simulink model "gtcs_math_magnetic_v0"  (R2022a)
settings: Solver=FixedStepDiscrete  StartTime=0.0  StopTime=10  FixedStep=1e-05  RelTol=1e-3
values from neighbouring files (symbols this model uses):
  B_r = 0.0001    [gtcs_math_magnetic_v0_dd.sldd]    (also in gtcs_math_magnetic_v0_parameter.mat)
  current_lim = 40.0    [gtcs_math_magnetic_v0_dd.sldd]    (also in gtcs_math_magnetic_v0_parameter.mat = 40)
  J_r = 0.00025    [gtcs_math_magnetic_v0_dd.sldd]    (also in gtcs_math_magnetic_v0_parameter.mat)
  L = 6.0E-6    [gtcs_math_magnetic_v0_dd.sldd]    (also in gtcs_math_magnetic_v0_parameter.mat = 6e-06)
  M = 3.0E-6    [gtcs_math_magnetic_v0_dd.sldd]    (also in gtcs_math_magnetic_v0_parameter.mat = 3e-06)
  P = 1.0    [gtcs_math_magnetic_v0_dd.sldd]    (also in gtcs_math_magnetic_v0_parameter.mat = 1)
  phase_a = 0.0    [gtcs_math_magnetic_v0_dd.sldd]    (also in gtcs_math_magnetic_v0_parameter.mat = 0)
  phase_b = 2.0943951023931953    [gtcs_math_magnetic_v0_dd.sldd]    (also in gtcs_math_magnetic_v0_parameter.mat = 2.09439510239)
  phase_c = -2.0943951023931953    [gtcs_math_magnetic_v0_dd.sldd]    (also in gtcs_math_magnetic_v0_parameter.mat = -2.09439510239)
  Phi_m = 0.04    [gtcs_math_magnetic_v0_dd.sldd]    (also in gtcs_math_magnetic_v0_parameter.mat)
  R = 0.015    [gtcs_math_magnetic_v0_dd.sldd]    (also in gtcs_math_magnetic_v0_parameter.mat)
undefined symbols (not defined in the file or in its folder): DiscIntNeverNeededParam
libraries: simulink x3
settings Model: DataDictionary=gtcs_math_magnetic_v0_dd.sldd  Creator=yusuf.ogut  LastModifiedBy=yusuf.ogut

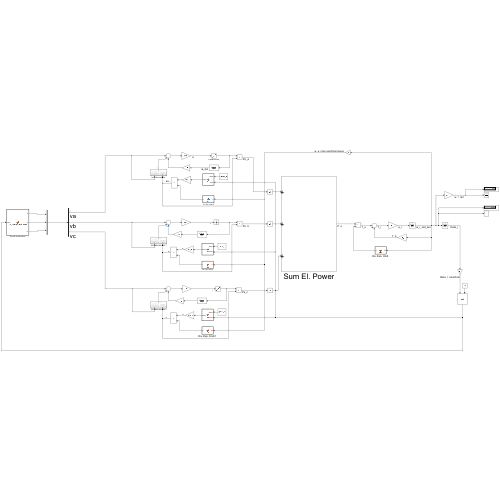
[thumbnail: Simulink's stored preview of the top-level diagram]
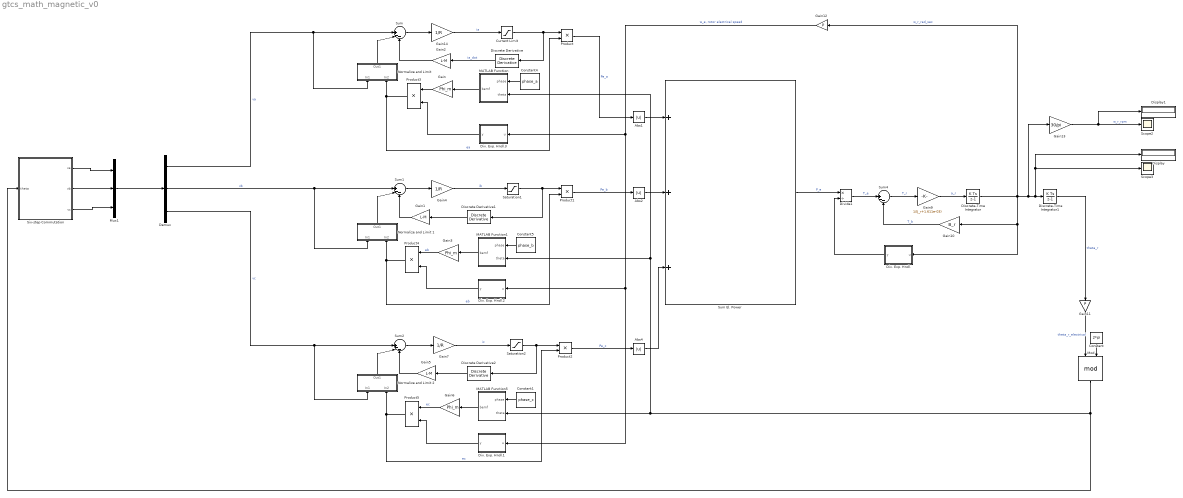
== system gtcs_math_magnetic_v0 ==
  Abs1 : Abs  SaturateOnIntegerOverflow=off
  Abs2 : Abs  SaturateOnIntegerOverflow=off
  Abs4 : Abs  SaturateOnIntegerOverflow=off
  Constant : Constant  Value=2*pi
  Constant1 : Constant  Value=phase_c
  Constant4 : Constant  Value=phase_a
  Constant5 : Constant  Value=phase_b
  Current Limit : Saturate  UpperLimit=current_lim  LowerLimit=-current_lim
  Demux : Demux  Outputs=3
  Discrete Derivative : simulink/Discrete/Discrete Derivative  gainval=1.0  ICPrevScaledInput=0.0  OutMin=[]  OutMax=[]  OutDataType=fixdt(1, 16)  OutScaling=2^-10  DoSatur=off
  Discrete Derivative1 : simulink/Discrete/Discrete Derivative  gainval=1.0  ICPrevScaledInput=0.0  OutMin=[]  OutMax=[]  OutDataType=fixdt(1, 16)  OutScaling=2^-10  DoSatur=off
  Discrete Derivative2 : simulink/Discrete/Discrete Derivative  gainval=1.0  ICPrevScaledInput=0.0  OutMin=[]  OutMax=[]  OutDataType=fixdt(1, 16)  OutScaling=2^-10  DoSatur=off
  Discrete-Time Integrator : DiscreteIntegrator  SampleTime=-1  ICPrevOutput=DiscIntNeverNeededParam  ICPrevScaledInput=DiscIntNeverNeededParam
  Discrete-Time Integrator1 : DiscreteIntegrator  SampleTime=-1  ICPrevOutput=DiscIntNeverNeededParam  ICPrevScaledInput=DiscIntNeverNeededParam
  Display : Display
  Display1 : Display
  Div. Exp. Hndl. : MATLAB Function  TreatAsAtomicUnit=on
  Div. Exp. Hndl.1 : MATLAB Function  TreatAsAtomicUnit=on
  Div. Exp. Hndl.2 : MATLAB Function  TreatAsAtomicUnit=on
  Div. Exp. Hndl.3 : MATLAB Function  TreatAsAtomicUnit=on
  Divide1 : Product  Inputs=*/
  Gain : Gain  Gain=Phi_m
  Gain1 : Gain  Gain=L-M
  Gain10 : Gain  Gain=B_r
  Gain11 : Gain  Gain=P
  Gain12 : Gain  Gain=P
  Gain13 : Gain  Gain=30/pi
  Gain14 : Gain  Gain=1/R
  Gain2 : Gain  Gain=L-M
  Gain3 : Gain  Gain=Phi_m
  Gain4 : Gain  Gain=1/R
  Gain5 : Gain  Gain=L-M
  Gain6 : Gain  Gain=Phi_m
  Gain7 : Gain  Gain=1/R
  Gain9 : Gain  Gain=1/(J_r+1.611e-03)
  MATLAB Function : MATLAB Function  TreatAsAtomicUnit=on
  MATLAB Function1 : MATLAB Function  TreatAsAtomicUnit=on
  MATLAB Function5 : MATLAB Function  TreatAsAtomicUnit=on
  Mod : Math  Operator=mod
  Mux1 : Mux  Inputs=3
  Normalize and Limit : Subsystem
  Normalize and Limit 1 : Subsystem
  Normalize and Limit 2 : Subsystem
  Product{,1..5} (6 alike) : Product
  Saturation1 : Saturate  UpperLimit=current_lim  LowerLimit=-current_lim
  Saturation2 : Saturate  UpperLimit=current_lim  LowerLimit=-current_lim
  Scope2 : Scope
  Scope3 : Scope
  Six-step Commutation : MATLAB Function  TreatAsAtomicUnit=on
  Sum{,1..2,4} (4 alike) : Sum  Inputs=||+--
  Sum El. Power : Sum  Inputs=+++
  wires:
  Demux/1 -> Sum/1, Normalize and Limit/1(In1)  "va"
  Gain14/1 -> Current Limit/1  "ia"
  Discrete Derivative/1 -> Gain2/1  "ia_dot"
  Product3/1 -> Normalize and Limit/2(In2), Product/2  "ea"
  Constant4/1 -> MATLAB Function/1(phase)
  Gain4/1 -> Saturation1/1  "ib"
  Constant5/1 -> MATLAB Function1/1(phase)
  Gain1/1 -> Sum1/3
  MATLAB Function1/1(bemf) -> Gain3/1
  Product4/1 -> Product1/2, Normalize and Limit 1/2(In2)  "eb"
  Demux/2 -> Sum1/1, Normalize and Limit 1/1(In1)  "vb"
  Sum1/1 -> Gain4/1
  Discrete Derivative1/1 -> Gain1/1
  MATLAB Function5/1(bemf) -> Gain6/1
  Demux/3 -> Sum2/1, Normalize and Limit 2/1(In1)  "vc"
  Product5/1 -> Normalize and Limit 2/2(In2), Product2/2  "ec"
  Discrete Derivative2/1 -> Gain5/1
  Gain5/1 -> Sum2/3
  Sum2/1 -> Gain7/1
  Gain7/1 -> Saturation2/1  "ic"
  Constant1/1 -> MATLAB Function5/1(phase)
  Sum4/1 -> Gain9/1  "T_r"
  Gain9/1 -> Discrete-Time Integrator/1  "a_r"
  Gain10/1 -> Sum4/3  "T_b"
  Discrete-Time Integrator/1 -> Gain12/1, Gain13/1, Scope3/1, Display/1, Discrete-Time Integrator1/1, Div. Exp. Hndl./1(u), Gain10/1  "w_r_rad_sec"
  Discrete-Time Integrator1/1 -> Gain11/1  "theta_r"
  Sum El. Power/1 -> Divide1/1  "P_e"
  Gain11/1 -> Mod/1  "theta_r_electrical"
  Constant/1 -> Mod/2
  Div. Exp. Hndl./1(y) -> Divide1/2
  Product/1 -> Abs1/1  "Pe_a"
  Divide1/1 -> Sum4/1  "T_e"
  Saturation1/1 -> Product1/1, Discrete Derivative1/1
  Saturation2/1 -> Discrete Derivative2/1, Product2/1
  Six-step Commutation/3(vc) -> Mux1/3
  Six-step Commutation/2(vb) -> Mux1/2
  Six-step Commutation/1(va) -> Mux1/1
  Mux1/1 -> Demux/1
  Gain12/1 -> Div. Exp. Hndl.3/1(u), Div. Exp. Hndl.1/1(u), Div. Exp. Hndl.2/1(u)  "w_e, rotor electrical speed"
  Gain/1 -> Product3/1
  Gain3/1 -> Product4/1  "eb"
  Gain6/1 -> Product5/1  "ec"
  Div. Exp. Hndl.3/1(y) -> Product3/2
  Div. Exp. Hndl.2/1(y) -> Product4/2
  Div. Exp. Hndl.1/1(y) -> Product5/2
  Gain13/1 -> Display1/1, Scope2/1  "w_r_rpm"
  Product1/1 -> Abs2/1  "Pe_b"
  Product2/1 -> Abs4/1  "Pe_c"
  Current Limit/1 -> Product/1, Discrete Derivative/1
  Normalize and Limit 1/1(Out1) -> Sum1/2
  Normalize and Limit 2/1(Out1) -> Sum2/2
  Normalize and Limit/1(Out1) -> Sum/2
  Sum/1 -> Gain14/1
  Abs1/1 -> Sum El. Power/1
  Abs2/1 -> Sum El. Power/2
  Mod/1 -> MATLAB Function5/2(theta), MATLAB Function1/2(theta), MATLAB Function/2(theta), Six-step Commutation/1(theta)
  Abs4/1 -> Sum El. Power/3
  Gain2/1 -> Sum/3
  MATLAB Function/1(bemf) -> Gain/1

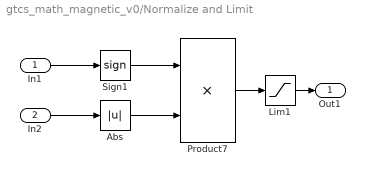
== system gtcs_math_magnetic_v0/Normalize and Limit ==
  In1 : Inport
  In2 : Inport  Port=2
  Abs : Abs  SaturateOnIntegerOverflow=off
  Lim1 : Saturate  UpperLimit=28  LowerLimit=-28
  Product7 : Product
  Sign1 : Signum
  Out1 : Outport
  wires:
  Lim1/1 -> Out1/1
  In2/1 -> Abs/1
  Sign1/1 -> Product7/1
  In1/1 -> Sign1/1
  Product7/1 -> Lim1/1
  Abs/1 -> Product7/2

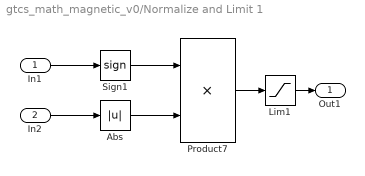
== system gtcs_math_magnetic_v0/Normalize and Limit 1 ==
  In1 : Inport
  In2 : Inport  Port=2
  Abs : Abs  SaturateOnIntegerOverflow=off
  Lim1 : Saturate  UpperLimit=28  LowerLimit=-28
  Product7 : Product
  Sign1 : Signum
  Out1 : Outport
  wires:
  Abs/1 -> Product7/2
  Product7/1 -> Lim1/1
  In1/1 -> Sign1/1
  Sign1/1 -> Product7/1
  In2/1 -> Abs/1
  Lim1/1 -> Out1/1

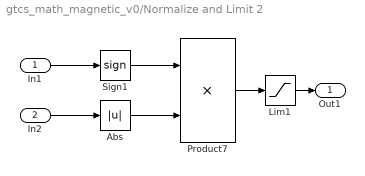
== system gtcs_math_magnetic_v0/Normalize and Limit 2 ==
  In1 : Inport
  In2 : Inport  Port=2
  Abs : Abs  SaturateOnIntegerOverflow=off
  Lim1 : Saturate  UpperLimit=28  LowerLimit=-28
  Product7 : Product
  Sign1 : Signum
  Out1 : Outport
  wires:
  Lim1/1 -> Out1/1
  In2/1 -> Abs/1
  Sign1/1 -> Product7/1
  In1/1 -> Sign1/1
  Product7/1 -> Lim1/1
  Abs/1 -> Product7/2

== matlab function gtcs_math_magnetic_v0/MATLAB Function ==
  data: phase input; bemf output; theta input
function bemf = fcn(phase, theta)
    theta_temp = mod(theta - phase,2*pi); % minus??
    bemf = 0;
    if theta_temp>=0 && theta_temp<(pi/6)
        %bemf = -theta_temp/(pi/6);
        bemf = -1;
    elseif theta_temp>=(pi/6) && theta_temp<(5*pi/6)
        bemf = -1;
    elseif theta_temp>=(5*pi/6) && theta_temp<(pi)
        %bemf = -1 + (theta_temp-5*pi/6)/(pi-5*pi/6);
        bemf = -1;
    elseif theta_temp>=(pi) && theta_temp<(7*pi/6)
        %bemf = (theta_temp-pi)/(7*pi/6-pi);
        bemf = 1;
    elseif theta_temp>=(7*pi/6) && theta_temp<(11*pi/6)
        bemf = 1;
    elseif theta_temp>=(11*pi/6) && theta_temp<(2*pi)
%         bemf = 1 - (theta_temp-11*pi/6)/(2*pi-11*pi/6);
        bemf = 1;
    end
end

== matlab function gtcs_math_magnetic_v0/Div. Exp. Hndl. ==
  data: u input; y output
function y = fcn(u)
    y = u;
    if u==0
        y = 999999999;
    end

== matlab function gtcs_math_magnetic_v0/Six-step Commutation ==
  data: theta input; va output; vb output; vc output
function [va, vb, vc] = fun_SixStepCommutation(theta)
    va = 0; vb = 0; vc = 0;
    theta = theta * 360 / 2 / pi;
    v_dclink = 28;
    if theta>=0 && theta<60
        va = 0; vb = v_dclink; vc = -v_dclink;
    elseif theta>=60 && theta<120
        va = v_dclink; vb = v_dclink; vc = 0;
    elseif theta>=120 && theta<180
        va = v_dclink; vb = 0; vc = v_dclink;
    elseif theta>=180 && theta<240
        va = 0; vb = -v_dclink; vc = v_dclink;
    elseif theta>=240 && theta<300
        va = - v_dclink; vb = -v_dclink; vc = 0;        
    elseif theta>=300 && theta<360
        va = - v_dclink; vb = 0; vc = -v_dclink;           
    end
end

== matlab function gtcs_math_magnetic_v0/Div. Exp. Hndl.3 ==
  data: u input; y output
function y = fcn(u)
    y = u;
    if u==0
        y = 0.1;
    end

end

== matlab function gtcs_math_magnetic_v0/Div. Exp. Hndl.2 ==
  data: u input; y output
function y = fcn(u)
    y = u;
    if u==0
        y = 0.1;
    end

end

== matlab function gtcs_math_magnetic_v0/Div. Exp. Hndl.1 ==
  data: u input; y output
function y = fcn(u)
    y = u;
    if u==0
        y = 0.1;
    end

end

== matlab function gtcs_math_magnetic_v0/MATLAB Function5 ==
  data: phase input; bemf output; theta input
function bemf = fcn(phase, theta)
    theta_temp = mod(theta - phase,2*pi); % minus??
    bemf = 0;
    if theta_temp>=0 && theta_temp<(pi/6)
        %bemf = -theta_temp/(pi/6);
        bemf = -1;
    elseif theta_temp>=(pi/6) && theta_temp<(5*pi/6)
        bemf = -1;
    elseif theta_temp>=(5*pi/6) && theta_temp<(pi)
        %bemf = -1 + (theta_temp-5*pi/6)/(pi-5*pi/6);
        bemf = -1;
    elseif theta_temp>=(pi) && theta_temp<(7*pi/6)
        %bemf = (theta_temp-pi)/(7*pi/6-pi);
        bemf = 1;
    elseif theta_temp>=(7*pi/6) && theta_temp<(11*pi/6)
        bemf = 1;
    elseif theta_temp>=(11*pi/6) && theta_temp<(2*pi)
%         bemf = 1 - (theta_temp-11*pi/6)/(2*pi-11*pi/6);
        bemf = 1;
    end
end

== matlab function gtcs_math_magnetic_v0/MATLAB Function1 ==
  data: phase input; bemf output; theta input
function bemf = fcn(phase, theta)
    theta_temp = mod(theta - phase,2*pi); % minus??
    bemf = 0;
    if theta_temp>=0 && theta_temp<(pi/6)
        %bemf = -theta_temp/(pi/6);
        bemf = -1;
    elseif theta_temp>=(pi/6) && theta_temp<(5*pi/6)
        bemf = -1;
    elseif theta_temp>=(5*pi/6) && theta_temp<(pi)
        %bemf = -1 + (theta_temp-5*pi/6)/(pi-5*pi/6);
        bemf = -1;
    elseif theta_temp>=(pi) && theta_temp<(7*pi/6)
        %bemf = (theta_temp-pi)/(7*pi/6-pi);
        bemf = 1;
    elseif theta_temp>=(7*pi/6) && theta_temp<(11*pi/6)
        bemf = 1;
    elseif theta_temp>=(11*pi/6) && theta_temp<(2*pi)
%         bemf = 1 - (theta_temp-11*pi/6)/(2*pi-11*pi/6);
        bemf = 1;
    end
end
